simulink model "TClabControlDT"  (R2026a)
settings: Solver=VariableStepAuto  StopTime=600
StartFcn:
  | reset_temp
values from neighbouring files (symbols this model uses):
  Cd = kp + ki*T*(z+1)/(2*(z-1))    [setupModelParametersDT.m]
  ki = 0.06    [setupModelParametersDT.m]    (also in setupModelParametersSat.m = 0.1)
  kp = 6.5    [setupModelParametersDT.m]    (also in setupModelParametersSat.m = 8.75)
  P = tf([-tau/2, 1],[tau/2 1])*tf(K,[1 a])    [setupModelParametersDT.m]    (also in setupModelParametersSat.m)
  T = 10    [setupModelParametersDT.m]
settings Model: Creator=jamess  LastModifiedBy=socks

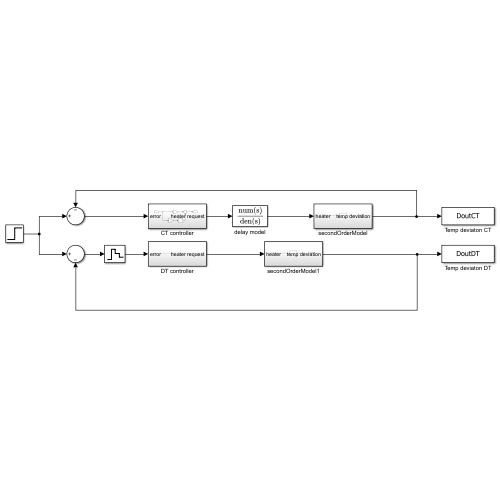
[thumbnail: Simulink's stored preview of the top-level diagram]
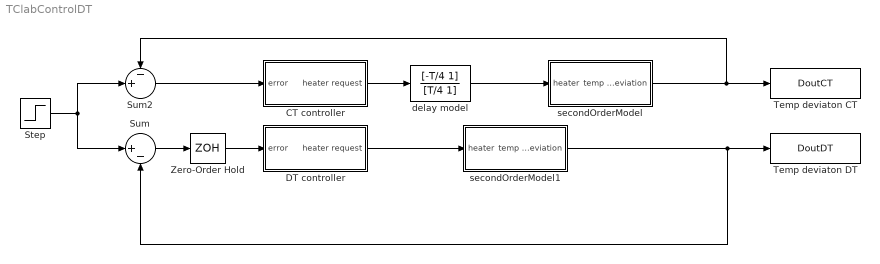
== system TClabControlDT ==
  CT controller : Subsystem
  DT controller : Subsystem
  Step : Step  Time=0  FinalValue=Dref  SampleTime=0
  Sum : Sum  Inputs=|+-
  Sum2 : Sum  Inputs=-+|
  Temp deviaton CT : ToWorkspace  VariableName=DoutCT  SaveFormat=Timeseries  SampleTime=-1
  Temp deviaton DT : ToWorkspace  VariableName=DoutDT  SaveFormat=Timeseries  SampleTime=-1
  Zero-Order Hold : ZeroOrderHold  SampleTime=T
  delay model : TransferFcn  Numerator=[-T/4 1]  Denominator=[T/4 1]
  secondOrderModel : Subsystem
  secondOrderModel1 : Subsystem
  wires:
  DT controller/1(heater request) -> secondOrderModel1/1(heater)
  Step/1 -> Sum/1, Sum2/2
  secondOrderModel1/1(temp deviation) -> Temp deviaton DT/1, Sum/2
  Sum/1 -> Zero-Order Hold/1
  Sum2/1 -> CT controller/1(error)
  Zero-Order Hold/1 -> DT controller/1(error)
  secondOrderModel/1(temp deviation) -> Temp deviaton CT/1, Sum2/1
  CT controller/1(heater request) -> delay model/1
  delay model/1 -> secondOrderModel/1(heater)

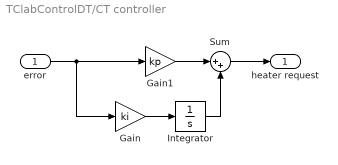
== system TClabControlDT/CT controller ==
  error : Inport
  Gain : Gain  Gain=ki
  Gain1 : Gain  Gain=kp
  Integrator : Integrator
  Sum : Sum  Inputs=|++
  heater request : Outport
  wires:
  error/1 -> Gain/1, Gain1/1
  Sum/1 -> heater request/1
  Gain/1 -> Integrator/1
  Gain1/1 -> Sum/1
  Integrator/1 -> Sum/2

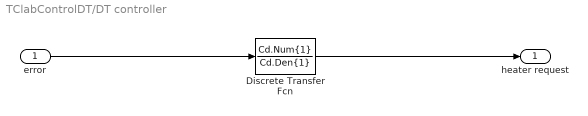
== system TClabControlDT/DT controller ==
  error : Inport
  Discrete Transfer Fcn : DiscreteTransferFcn  Numerator=Cd.Num{1}  Denominator=Cd.Den{1}  SampleTime=T
  heater request : Outport
  wires:
  error/1 -> Discrete Transfer Fcn/1
  Discrete Transfer Fcn/1 -> heater request/1

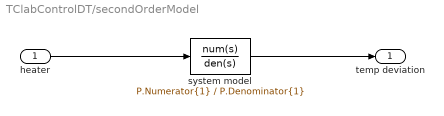
== system TClabControlDT/secondOrderModel ==
  heater : Inport
  system model : TransferFcn  Numerator=P.Numerator{1}  Denominator=P.Denominator{1}
  temp deviation : Outport
  wires:
  heater/1 -> system model/1
  system model/1 -> temp deviation/1

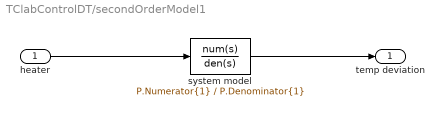
== system TClabControlDT/secondOrderModel1 ==
  heater : Inport
  system model : TransferFcn  Numerator=P.Numerator{1}  Denominator=P.Denominator{1}
  temp deviation : Outport
  wires:
  heater/1 -> system model/1
  system model/1 -> temp deviation/1
